simulink model "ChiefMaster_TTC580"  (R2022b)
settings: Solver=FixedStepAuto  StartTime=0.0  StopTime=10  FixedStep=0.01  RelTol=1e-3
values from neighbouring files (symbols this model uses):
  BattBox1_No = single(1)    [Parameters.m]
  BattBox2_No = single(2)    [Parameters.m]
  BattBox3_No = single(3)    [Parameters.m]
  CurrentLB = single(-3)    [Parameters.m]
  CurrentReductionConstant_Lvl0 = single(0.03)    [Parameters.m]
  CurrentReductionConstant_Lvl1 = single(0.05)    [Parameters.m]
  CurrentReductionConstant_Lvl2 = single(0.07)    [Parameters.m]
  CurrentReductionConstant_Lvl3 = single(0.1)    [Parameters.m]
  CurrentUB = single(3)    [Parameters.m]
  DCHV_Minus_In_Delay_ms = single(500)    [Parameters.m]
  FL_sHVC_CellBalanceVoltage_mV = single(3500)    [Parameters.m]
  FL_sInrushCurrent_dividebyzero = single(0.00001)    [Parameters.m]
  FL_u8HMI_BuzzerTimer = uint8(3)    [Parameters.m]
  IP_boActValue = true    [Parameters.m]
  IP_boDeactValue = false    [Parameters.m]
  IP_boInitValue = false    [Parameters.m]
  IP_s_LB = 18000    [Parameters.m]
  IP_s_UB = 22000    [Parameters.m]
  IP_sBatt1_ChargeCurrentMax_Factor = single(0.1)    [Parameters.m]
  IP_sBatt1_ChargeCurrentMax_LB = single(0)    [Parameters.m]
  IP_sBatt1_ChargeCurrentMax_Offset = single(0)    [Parameters.m]
  IP_sBatt1_ChargeCurrentMax_UB = single(6553.5)    [Parameters.m]
  IP_sBatt1_Current_Factor = single(0.1)    [Parameters.m]
  IP_sBatt1_Current_LB = single(-3276.8)    [Parameters.m]
  IP_sBatt1_Current_Offset = single(0)    [Parameters.m]
  IP_sBatt1_Current_UB = single(3276.8)    [Parameters.m]
  IP_sBatt1_DisChargeCurrentMax_Factor = single(0.1)    [Parameters.m]
  IP_sBatt1_DisChargeCurrentMax_LB = single(0)    [Parameters.m]
  IP_sBatt1_DisChargeCurrentMax_Offset = single(0)    [Parameters.m]
  IP_sBatt1_DisChargeCurrentMax_UB = single(6553.5)    [Parameters.m]
  IP_sBatt1_InsulationResistance_Factor = single(5)    [Parameters.m]
  IP_sBatt1_InsulationResistance_LB = single(0)    [Parameters.m]
  IP_sBatt1_InsulationResistance_Offset = single(0)    [Parameters.m]
  IP_sBatt1_InsulationResistance_UB = single(0)    [Parameters.m]
  IP_sBatt1_LiBa_IntResist_mOhm = single(25)    [Parameters.m]
  IP_sBatt1_SOC_Factor = single(1)    [Parameters.m]
  IP_sBatt1_SOC_LB = single(0)    [Parameters.m]
  IP_sBatt1_SOC_Offset = single(0)    [Parameters.m]
  IP_sBatt1_SOC_UB = single(100)    [Parameters.m]
  IP_sBatt1_SOH_Factor = single(1)    [Parameters.m]
  IP_sBatt1_SOH_LB = single(0)    [Parameters.m]
  IP_sBatt1_SOH_Offset = single(0)    [Parameters.m]
  IP_sBatt1_SOH_UB = single(100)    [Parameters.m]
  IP_sBatt1_Ubatt_Factor = single(0.1)    [Parameters.m]
  IP_sBatt1_Ubatt_LB = single(0)    [Parameters.m]
  IP_sBatt1_Ubatt_Offset = single(0)    [Parameters.m]
  IP_sBatt1_Ubatt_UB = single(6553.5)    [Parameters.m]
  IP_sBatt1_UserRi_Factor = single(1)    [Parameters.m]
  IP_sBatt1_UserRi_LB = single(0)    [Parameters.m]
  IP_sBatt1_UserRi_Offset = single(0)    [Parameters.m]
  IP_sBatt1_UserRi_UB = single(255)    [Parameters.m]
  IP_sBatt1_VoltageAtSensor_Factor = single(0.02)    [Parameters.m]
  IP_sBatt1_VoltageAtSensor_LB = single(0)    [Parameters.m]
  IP_sBatt1_VoltageAtSensor_Offset = single(0)    [Parameters.m]
  IP_sBatt1_VoltageAtSensor_UB = single(1310.7)    [Parameters.m]
  IP_sBatt2_LiBa_IntResist_mOhm = single(25)    [Parameters.m]
  IP_sBatt3_LiBa_IntResist_mOhm = single(25)    [Parameters.m]
  IP_sEM_LB = 2000    [Parameters.m]
  IP_sEM_UB = 8000    [Parameters.m]
  IP_sFB_LB = 5000    [Parameters.m]
  IP_sFB_UB = 10000    [Parameters.m]
  IP_sHVIL_LB = 12000    [Parameters.m]
  IP_sHVIL_UB = 15000    [Parameters.m]
  IP_sLoad_Voltage_Factor = single(1)    [Parameters.m]
  IP_sLoad_Voltage_LB = single(0)    [Parameters.m]
  IP_sLoad_Voltage_Offset = single(0)    [Parameters.m]
  IP_sLoad_Voltage_UB = single(65535)    [Parameters.m]
  IP_u8HVIL_Delay_ms = uint8(100)    [Parameters.m]
  IP_u8HW_IN_delay_ms = uint8(100)    [Parameters.m]
  IT_sInsulationSafeValue_kOhm = single(650)    [Parameters.m]
  IT_u8IMD_DelayTime_s = uint8(20)    [Parameters.m]
  MainHV_Minus_In_Delay = single(5)    [Parameters.m]
  MainHV_StatusDelay = single(5)    [Parameters.m]
  NotAvailable_uint16 = single(65535)    [Parameters.m]
  NotAvailable_uint8 = uint8(255)    [Parameters.m]
  OP_boHVIL_Supply = boolean(1)    [Parameters.m]
  SafeCurrentToCloseHV_A = single(5)    [Parameters.m]
  SafeVoltageToCloseHV_V = single(0.5)    [Parameters.m]
  UnexpectedBattChargingFcn_Available = boolean(1)    [Parameters.m]
  Voltage_NA_UB = uint16(65535)    [Parameters.m]
  VoltageSensorAvailableBB1 = boolean(0)    [Parameters.m]
  VoltageSensorAvailableBB2 = boolean(0)    [Parameters.m]
  VoltageSensorAvailableBB3 = boolean(0)    [Parameters.m]
libraries: simulink x184, Library_DataProcessing_v1_1 x167, Library_DataProcessing_v1 x142, libCM x28
(part 2 of 19)

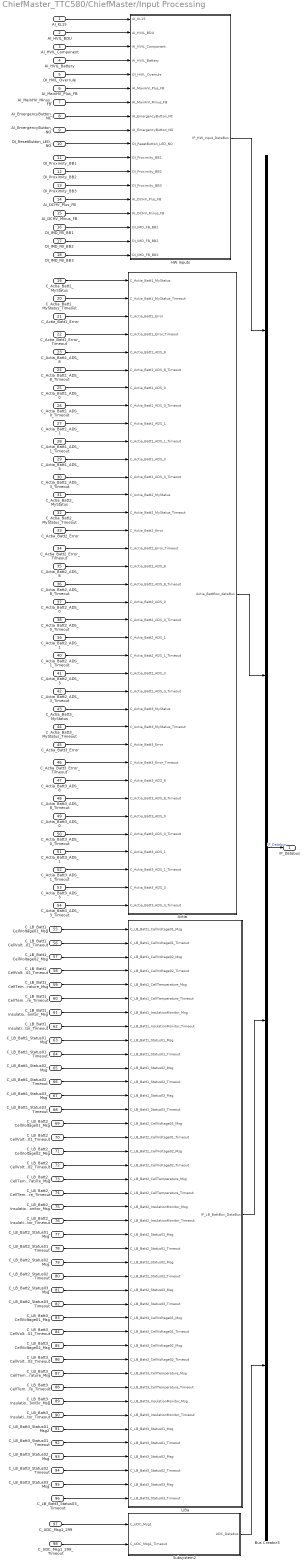
== system ChiefMaster_TTC580/ChiefMaster/Input Processing ==
  AI_KL15 : Inport  OutDataTypeStr=single
  AI_HVIL_BDU : Inport  Port=2  OutDataTypeStr=single
  AI_HVIL_Component : Inport  Port=3  OutDataTypeStr=single
  AI_HVIL_Battery : Inport  Port=4  OutDataTypeStr=single
  DI_HVIL_Overrule : Inport  Port=5  OutDataTypeStr=boolean
  AI_MainHV_Plus_FB : Inport  Port=6  OutDataTypeStr=single
  AI_MainHV_Minus_FB : Inport  Port=7  OutDataTypeStr=single
  AI_EmergencyButton_NC : Inport  Port=8  OutDataTypeStr=single
  AI_EmergencyButton_NO : Inport  Port=9
  DI_ResetButton_LED_NO : Inport  Port=10
  DI_Proximity_BB1 : Inport  Port=11
  DI_Proximity_BB2 : Inport  Port=12
  DI_Proximity_BB3 : Inport  Port=13
  AI_DCHV_Plus_FB : Inport  Port=14  OutDataTypeStr=single
  AI_DCHV_Minus_FB : Inport  Port=15  OutDataTypeStr=single
  DI_IMD_FB_BB1 : Inport  Port=16
  DI_IMD_FB_BB2 : Inport  Port=17
  DI_IMD_FB_BB3 : Inport  Port=18
  C_Actia_Batt1_MyStatus : Inport  Port=19  OutDataTypeStr=uint8
  C_Actia_Batt1_MyStatus_Timeout : Inport  Port=20  OutDataTypeStr=boolean
  C_Actia_Batt1_Error : Inport  Port=21  OutDataTypeStr=uint8
  C_Actia_Batt1_Error_Timeout : Inport  Port=22  OutDataTypeStr=boolean
  C_Actia_Batt1_ADS_8 : Inport  Port=23  OutDataTypeStr=uint8
  C_Actia_Batt1_ADS_8_Timeout : Inport  Port=24  OutDataTypeStr=boolean
  C_Actia_Batt1_ADS_0 : Inport  Port=25
  C_Actia_Batt1_ADS_0_Timeout : Inport  Port=26
  C_Actia_Batt1_ADS_1 : Inport  Port=27  OutDataTypeStr=uint8
  C_Actia_Batt1_ADS_1_Timeout : Inport  Port=28  OutDataTypeStr=boolean
  C_Actia_Batt1_ADS_3 : Inport  Port=29  OutDataTypeStr=uint8
  C_Actia_Batt1_ADS_3_Timeout : Inport  Port=30  OutDataTypeStr=boolean
  C_Actia_Batt2_MyStatus : Inport  Port=31  OutDataTypeStr=uint8
  C_Actia_Batt2_MyStatus_Timeout : Inport  Port=32  OutDataTypeStr=boolean
  C_Actia_Batt2_Error : Inport  Port=33  OutDataTypeStr=uint8
  C_Actia_Batt2_Error_Timeout : Inport  Port=34  OutDataTypeStr=boolean
  C_Actia_Batt2_ADS_8 : Inport  Port=35  OutDataTypeStr=uint8
  C_Actia_Batt2_ADS_8_Timeout : Inport  Port=36  OutDataTypeStr=boolean
  C_Actia_Batt2_ADS_0 : Inport  Port=37
  C_Actia_Batt2_ADS_0_Timeout : Inport  Port=38
  C_Actia_Batt2_ADS_1 : Inport  Port=39  OutDataTypeStr=uint8
  C_Actia_Batt2_ADS_1_Timeout : Inport  Port=40  OutDataTypeStr=boolean
  C_Actia_Batt2_ADS_3 : Inport  Port=41  OutDataTypeStr=uint8
  C_Actia_Batt2_ADS_3_Timeout : Inport  Port=42  OutDataTypeStr=boolean
  C_Actia_Batt3_MyStatus : Inport  Port=43  OutDataTypeStr=uint8
  C_Actia_Batt3_MyStatus_Timeout : Inport  Port=44  OutDataTypeStr=boolean
  C_Actia_Batt3_Error : Inport  Port=45  OutDataTypeStr=uint8
  C_Actia_Batt3_Error_Timeout : Inport  Port=46  OutDataTypeStr=boolean
  C_Actia_Batt3_ADS_8 : Inport  Port=47  OutDataTypeStr=uint8
  C_Actia_Batt3_ADS_8_Timeout : Inport  Port=48  OutDataTypeStr=boolean
  C_Actia_Batt3_ADS_0 : Inport  Port=49
  C_Actia_Batt3_ADS_0_Timeout : Inport  Port=50
  C_Actia_Batt3_ADS_1 : Inport  Port=51  OutDataTypeStr=uint8
  C_Actia_Batt3_ADS_1_Timeout : Inport  Port=52  OutDataTypeStr=boolean
  C_Actia_Batt3_ADS_3 : Inport  Port=53  OutDataTypeStr=uint8
  C_Actia_Batt3_ADS_3_Timeout : Inport  Port=54  OutDataTypeStr=boolean
  C_LB_Batt1_CellVoltage01_Msg : Inport  Port=55
  C_LB_Batt1_CellVoltage01_Timeout : Inport  Port=56
  C_LB_Batt1_CellVoltage02_Msg : Inport  Port=57
  C_LB_Batt1_CellVoltage02_Timeout : Inport  Port=58
  C_LB_Batt1_CellTemperature_Msg : Inport  Port=59
  C_LB_Batt1_CellTemperature_Timeout : Inport  Port=60
  C_LB_Batt1_InsulationMonitor_Msg : Inport  Port=61
  C_LB_Batt1_InsulationMonitor_Timeout : Inport  Port=62
  C_LB_Batt1_Status01_Msg : Inport  Port=63
  C_LB_Batt1_Status01_Timeout : Inport  Port=64
  C_LB_Batt1_Status02_Msg : Inport  Port=65
  C_LB_Batt1_Status02_Timeout : Inport  Port=66
  C_LB_Batt1_Status03_Msg : Inport  Port=67
  C_LB_Batt1_Status03_Timeout : Inport  Port=68
  C_LB_Batt2_CellVoltage01_Msg : Inport  Port=69
  C_LB_Batt2_CellVoltage01_Timeout : Inport  Port=70
  C_LB_Batt2_CellVoltage02_Msg : Inport  Port=71
  C_LB_Batt2_CellVoltage02_Timeout : Inport  Port=72
  C_LB_Batt2_CellTemperature_Msg : Inport  Port=73
  C_LB_Batt2_CellTemperature_Timeout : Inport  Port=74
  C_LB_Batt2_InsulationMonitor_Msg : Inport  Port=75
  C_LB_Batt2_InsulationMonitor_Timeout : Inport  Port=76
  C_LB_Batt2_Status01_Msg : Inport  Port=77
  C_LB_Batt2_Status01_Timeout : Inport  Port=78
  C_LB_Batt2_Status02_Msg : Inport  Port=79
  C_LB_Batt2_Status02_Timeout : Inport  Port=80
  C_LB_Batt2_Status03_Msg : Inport  Port=81
  C_LB_Batt2_Status03_Timeout : Inport  Port=82
  C_LB_Batt3_CellVoltage01_Msg : Inport  Port=83
  C_LB_Batt3_CellVoltage01_Timeout : Inport  Port=84
  C_LB_Batt3_CellVoltage02_Msg : Inport  Port=85
  C_LB_Batt3_CellVoltage02_Timeout : Inport  Port=86
  C_LB_Batt3_CellTemperature_Msg : Inport  Port=87
  C_LB_Batt3_CellTemperature_Timeout : Inport  Port=88
  C_LB_Batt3_InsulationMonitor_Msg : Inport  Port=89
  C_LB_Batt3_InsulationMonitor_Timeout : Inport  Port=90
  C_LB_Batt3_Status01_Msg2 : Inport  Port=91
  C_LB_Batt3_Status01_Timeout : Inport  Port=92
  C_LB_Batt3_Status02_Msg : Inport  Port=93
  C_LB_Batt3_Status02_Timeout : Inport  Port=94
  C_LB_Batt3_Status03_Msg : Inport  Port=95
  C_LB_Batt3_Status03_Timeout : Inport  Port=96
  C_UDC_Msg1_299 : Inport  Port=97
  C_UDC_Msg1_299_Timeout : Inport  Port=98
  Actia : Subsystem
  Bus Creator3 : BusCreator  Inputs=4
  HW Inputs : Subsystem
  LiBa : Subsystem
  Subsystem2 : Subsystem
  IP_Databus : Outport
  wires:
  AI_MainHV_Minus_FB/1 -> HW Inputs/7(AI_MainHV_Minus_FB)
  AI_KL15/1 -> HW Inputs/1(AI_KL15)
  AI_MainHV_Plus_FB/1 -> HW Inputs/6(AI_MainHV_Plus_FB)
  Bus Creator3/1 -> IP_Databus/1  "IP_Databus"
  Subsystem2/1(UDC_Databus) -> Bus Creator3/4
  C_LB_Batt1_CellVoltage02_Msg/1 -> LiBa/3(C_LB_Batt1_CellVoltage02_Msg)
  C_LB_Batt1_CellVoltage01_Timeout/1 -> LiBa/2(C_LB_Batt1_CellVoltage01_Timeout)
  C_LB_Batt1_CellVoltage01_Msg/1 -> LiBa/1(C_LB_Batt1_CellVoltage01_Msg)
  C_LB_Batt1_InsulationMonitor_Msg/1 -> LiBa/7(C_LB_Batt1_InsulationMonitor_Msg)
  C_LB_Batt1_CellTemperature_Timeout/1 -> LiBa/6(C_LB_Batt1_CellTemperature_Timeout)
  C_LB_Batt1_CellTemperature_Msg/1 -> LiBa/5(C_LB_Batt1_CellTemperature_Msg)
  C_LB_Batt1_CellVoltage02_Timeout/1 -> LiBa/4(C_LB_Batt1_CellVoltage02_Timeout)
  C_UDC_Msg1_299/1 -> Subsystem2/1(C_UDC_Msg1)
  C_LB_Batt1_Status02_Msg/1 -> LiBa/11(C_LB_Batt1_Status02_Msg)
  C_LB_Batt1_Status01_Timeout/1 -> LiBa/10(C_LB_Batt1_Status01_Timeout)
  C_LB_Batt1_Status01_Msg/1 -> LiBa/9(C_LB_Batt1_Status01_Msg)
  C_LB_Batt1_InsulationMonitor_Timeout/1 -> LiBa/8(C_LB_Batt1_InsulationMonitor_Timeout)
  C_LB_Batt1_Status03_Timeout/1 -> LiBa/14(C_LB_Batt1_Status03_Timeout)
  C_LB_Batt1_Status03_Msg/1 -> LiBa/13(C_LB_Batt1_Status03_Msg)
  C_LB_Batt1_Status02_Timeout/1 -> LiBa/12(C_LB_Batt1_Status02_Timeout)
  C_UDC_Msg1_299_Timeout/1 -> Subsystem2/2(C_UDC_Msg1_Timeout)
  HW Inputs/1(IP_HW_Input_DataBus) -> Bus Creator3/1
  Actia/1(Actia_BattBox_dataBus) -> Bus Creator3/2
  C_LB_Batt3_Status03_Timeout/1 -> LiBa/42(C_LB_Batt3_Status03_Timeout)
  C_LB_Batt3_CellVoltage02_Msg/1 -> LiBa/31(C_LB_Batt3_CellVoltage02_Msg)
  C_LB_Batt3_InsulationMonitor_Timeout/1 -> LiBa/36(C_LB_Batt3_InsulationMonitor_Timeout)
  C_LB_Batt3_CellVoltage02_Timeout/1 -> LiBa/32(C_LB_Batt3_CellVoltage02_Timeout)
  C_LB_Batt3_CellVoltage01_Timeout/1 -> LiBa/30(C_LB_Batt3_CellVoltage01_Timeout)
  C_LB_Batt3_Status01_Msg2/1 -> LiBa/37(C_LB_Batt3_Status01_Msg)
  C_LB_Batt3_Status02_Timeout/1 -> LiBa/40(C_LB_Batt3_Status02_Timeout)
  C_LB_Batt3_Status02_Msg/1 -> LiBa/39(C_LB_Batt3_Status02_Msg)
  C_LB_Batt3_CellTemperature_Timeout/1 -> LiBa/34(C_LB_Batt3_CellTemperature_Timeout)
  C_LB_Batt3_Status03_Msg/1 -> LiBa/41(C_LB_Batt3_Status03_Msg)
  C_LB_Batt3_CellTemperature_Msg/1 -> LiBa/33(C_LB_Batt3_CellTemperature_Msg)
  C_LB_Batt3_InsulationMonitor_Msg/1 -> LiBa/35(C_LB_Batt3_InsulationMonitor_Msg)
  C_LB_Batt2_Status02_Timeout/1 -> LiBa/26(C_LB_Batt2_Status02_Timeout)
  C_LB_Batt2_Status03_Timeout/1 -> LiBa/28(C_LB_Batt2_Status03_Timeout)
  C_LB_Batt3_Status01_Timeout/1 -> LiBa/38(C_LB_Batt3_Status01_Timeout)
  C_LB_Batt2_Status03_Msg/1 -> LiBa/27(C_LB_Batt2_Status03_Msg)
  C_LB_Batt2_Status01_Timeout/1 -> LiBa/24(C_LB_Batt2_Status01_Timeout)
  C_LB_Batt2_Status01_Msg/1 -> LiBa/23(C_LB_Batt2_Status01_Msg)
  C_LB_Batt2_InsulationMonitor_Timeout/1 -> LiBa/22(C_LB_Batt2_InsulationMonitor_Timeout)
  C_LB_Batt2_CellVoltage02_Msg/1 -> LiBa/17(C_LB_Batt2_CellVoltage02_Msg)
  C_LB_Batt2_CellVoltage01_Timeout/1 -> LiBa/16(C_LB_Batt2_CellVoltage01_Timeout)
  C_LB_Batt2_InsulationMonitor_Msg/1 -> LiBa/21(C_LB_Batt2_InsulationMonitor_Msg)
  C_LB_Batt2_CellTemperature_Timeout/1 -> LiBa/20(C_LB_Batt2_CellTemperature_Timeout)
  C_LB_Batt2_CellVoltage02_Timeout/1 -> LiBa/18(C_LB_Batt2_CellVoltage02_Timeout)
  C_LB_Batt2_Status02_Msg/1 -> LiBa/25(C_LB_Batt2_Status02_Msg)
  C_LB_Batt2_CellTemperature_Msg/1 -> LiBa/19(C_LB_Batt2_CellTemperature_Msg)
  C_LB_Batt2_CellVoltage01_Msg/1 -> LiBa/15(C_LB_Batt2_CellVoltage01_Msg)
  C_LB_Batt3_CellVoltage01_Msg/1 -> LiBa/29(C_LB_Batt3_CellVoltage01_Msg)
  LiBa/1(IP_LB_BattBox_DataBus) -> Bus Creator3/3
  AI_HVIL_Battery/1 -> HW Inputs/4(AI_HVIL_Battery)
  AI_HVIL_Component/1 -> HW Inputs/3(AI_HVIL_Component)
  AI_HVIL_BDU/1 -> HW Inputs/2(AI_HVIL_BDU)
  AI_EmergencyButton_NC/1 -> HW Inputs/8(AI_EmergencyButton_NC)
  AI_EmergencyButton_NO/1 -> HW Inputs/9(AI_EmergencyButton_NO)
  DI_ResetButton_LED_NO/1 -> HW Inputs/10(DI_ResetButton_LED_NO)
  DI_Proximity_BB1/1 -> HW Inputs/11(DI_Proximity_BB1)
  DI_Proximity_BB2/1 -> HW Inputs/12(DI_Proximity_BB2)
  DI_Proximity_BB3/1 -> HW Inputs/13(DI_Proximity_BB3)
  AI_DCHV_Plus_FB/1 -> HW Inputs/14(AI_DCHV_Plus_FB)
  AI_DCHV_Minus_FB/1 -> HW Inputs/15(AI_DCHV_Minus_FB)
  C_Actia_Batt1_MyStatus/1 -> Actia/1(C_Actia_Batt1_MyStatus)
  C_Actia_Batt1_MyStatus_Timeout/1 -> Actia/2(C_Actia_Batt1_MyStatus_Timeout)
  C_Actia_Batt1_Error/1 -> Actia/3(C_Actia_Batt1_Error)
  C_Actia_Batt1_Error_Timeout/1 -> Actia/4(C_Actia_Batt1_Error_Timeout)
  C_Actia_Batt1_ADS_8/1 -> Actia/5(C_Actia_Batt1_ADS_8)
  C_Actia_Batt1_ADS_8_Timeout/1 -> Actia/6(C_Actia_Batt1_ADS_8_Timeout)
  C_Actia_Batt1_ADS_1/1 -> Actia/9(C_Actia_Batt1_ADS_1)
  C_Actia_Batt1_ADS_1_Timeout/1 -> Actia/10(C_Actia_Batt1_ADS_1_Timeout)
  C_Actia_Batt1_ADS_3/1 -> Actia/11(C_Actia_Batt1_ADS_3)
  C_Actia_Batt1_ADS_3_Timeout/1 -> Actia/12(C_Actia_Batt1_ADS_3_Timeout)
  C_Actia_Batt2_MyStatus/1 -> Actia/13(C_Actia_Batt2_MyStatus)
  C_Actia_Batt2_MyStatus_Timeout/1 -> Actia/14(C_Actia_Batt2_MyStatus_Timeout)
  C_Actia_Batt2_Error/1 -> Actia/15(C_Actia_Batt2_Error)
  C_Actia_Batt2_Error_Timeout/1 -> Actia/16(C_Actia_Batt2_Error_Timeout)
  C_Actia_Batt2_ADS_8/1 -> Actia/17(C_Actia_Batt2_ADS_8)
  C_Actia_Batt2_ADS_8_Timeout/1 -> Actia/18(C_Actia_Batt2_ADS_8_Timeout)
  C_Actia_Batt2_ADS_1/1 -> Actia/21(C_Actia_Batt2_ADS_1)
  C_Actia_Batt2_ADS_1_Timeout/1 -> Actia/22(C_Actia_Batt2_ADS_1_Timeout)
  C_Actia_Batt2_ADS_3/1 -> Actia/23(C_Actia_Batt2_ADS_3)
  C_Actia_Batt2_ADS_3_Timeout/1 -> Actia/24(C_Actia_Batt2_ADS_3_Timeout)
  C_Actia_Batt3_MyStatus/1 -> Actia/25(C_Actia_Batt3_MyStatus)
  C_Actia_Batt3_MyStatus_Timeout/1 -> Actia/26(C_Actia_Batt3_MyStatus_Timeout)
  C_Actia_Batt3_Error/1 -> Actia/27(C_Actia_Batt3_Error)
  C_Actia_Batt3_Error_Timeout/1 -> Actia/28(C_Actia_Batt3_Error_Timeout)
  C_Actia_Batt3_ADS_8/1 -> Actia/29(C_Actia_Batt3_ADS_8)
  C_Actia_Batt3_ADS_8_Timeout/1 -> Actia/30(C_Actia_Batt3_ADS_8_Timeout)
  C_Actia_Batt3_ADS_1/1 -> Actia/33(C_Actia_Batt3_ADS_1)
  C_Actia_Batt3_ADS_1_Timeout/1 -> Actia/34(C_Actia_Batt3_ADS_1_Timeout)
  C_Actia_Batt3_ADS_3/1 -> Actia/35(C_Actia_Batt3_ADS_3)
  C_Actia_Batt3_ADS_3_Timeout/1 -> Actia/36(C_Actia_Batt3_ADS_3_Timeout)
  C_Actia_Batt1_ADS_0_Timeout/1 -> Actia/8(C_Actia_Batt1_ADS_0_Timeout)
  C_Actia_Batt1_ADS_0/1 -> Actia/7(C_Actia_Batt1_ADS_0)
  C_Actia_Batt2_ADS_0/1 -> Actia/19(C_Actia_Batt2_ADS_0)
  C_Actia_Batt2_ADS_0_Timeout/1 -> Actia/20(C_Actia_Batt2_ADS_0_Timeout)
  C_Actia_Batt3_ADS_0_Timeout/1 -> Actia/32(C_Actia_Batt3_ADS_0_Timeout)
  C_Actia_Batt3_ADS_0/1 -> Actia/31(C_Actia_Batt3_ADS_0)
  DI_HVIL_Overrule/1 -> HW Inputs/5(DI_HVIL_Overrule)
  DI_IMD_FB_BB1/1 -> HW Inputs/16(DI_IMD_FB_BB1)
  DI_IMD_FB_BB2/1 -> HW Inputs/17(DI_IMD_FB_BB2)
  DI_IMD_FB_BB3/1 -> HW Inputs/18(DI_IMD_FB_BB3)

== system ChiefMaster_TTC580/ChiefMaster/Input Translation ==
  IP_Databus : Inport
  IMD_Req_Databus : Inport  Port=2
  Battery Selection : Subsystem
      settings: RTWFcnNameOpts=Use subsystem name  RTWFileNameOpts=Use subsystem name
  Battery Signals : Subsystem
  Bus Creator : BusCreator  Inputs=4
  HW Inputs : Subsystem
  UDC : Subsystem
  IT_Databus : Outport
  wires:
  IMD_Req_Databus/1 -> Battery Signals/2(IMD_Req_Databus)
  Battery Signals/1(IT_BatterySignal_Databus) -> Bus Creator/3
  Bus Creator/1 -> IT_Databus/1  "IT_Databus"
  HW Inputs/1(IT_HW_Input_Databus) -> Bus Creator/2
  UDC/1(IT_UDC_Databus) -> Bus Creator/4
  IP_Databus/1 -> UDC/1(IP_Databus), Battery Signals/1(IP_Databus), Battery Selection/1(IP_Databus), HW Inputs/1(IP_Databus)
  Battery Selection/1(IT_SelectBattery_Databus) -> Bus Creator/1

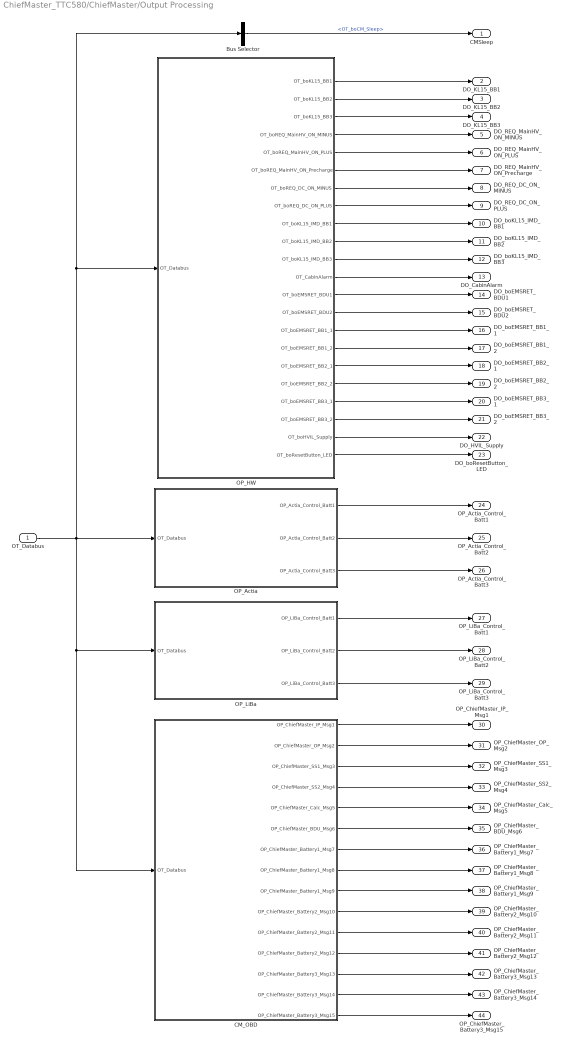
== system ChiefMaster_TTC580/ChiefMaster/Output Processing ==
  OT_Databus : Inport
  Bus Selector : BusSelector  OutputSignals=OT_boCM_Sleep
  CM_OBD : Subsystem
  OP_Actia : Subsystem
  OP_HW : Subsystem
  OP_LiBa : Subsystem
  CMSleep : Outport
  DO_KL15_BB1 : Outport  Port=2
  DO_KL15_BB2 : Outport  Port=3
  DO_KL15_BB3 : Outport  Port=4
  DO_REQ_MainHV_ON_MINUS : Outport  Port=5
  DO_REQ_MainHV_ON_PLUS : Outport  Port=6
  DO_REQ_MainHV_ON_Precharge : Outport  Port=7
  DO_REQ_DC_ON_MINUS : Outport  Port=8
  DO_REQ_DC_ON_PLUS : Outport  Port=9
  DO_boKL15_IMD_BB1 : Outport  Port=10
  DO_boKL15_IMD_BB2 : Outport  Port=11
  DO_boKL15_IMD_BB3 : Outport  Port=12
  DO_CabinAlarm : Outport  Port=13
  DO_boEMSRET_BDU1 : Outport  Port=14  OutDataTypeStr=boolean
  DO_boEMSRET_BDU2 : Outport  Port=15  OutDataTypeStr=boolean
  DO_boEMSRET_BB1_1 : Outport  Port=16  OutDataTypeStr=boolean
  DO_boEMSRET_BB1_2 : Outport  Port=17  OutDataTypeStr=boolean
  DO_boEMSRET_BB2_1 : Outport  Port=18  OutDataTypeStr=boolean
  DO_boEMSRET_BB2_2 : Outport  Port=19  OutDataTypeStr=boolean
  DO_boEMSRET_BB3_1 : Outport  Port=20  OutDataTypeStr=boolean
  DO_boEMSRET_BB3_2 : Outport  Port=21  OutDataTypeStr=boolean
  DO_HVIL_Supply : Outport  Port=22  OutDataTypeStr=boolean
  DO_boResetButton_LED : Outport  Port=23  OutDataTypeStr=boolean
  OP_Actia_Control_Batt1 : Outport  Port=24
  OP_Actia_Control_Batt2 : Outport  Port=25
  OP_Actia_Control_Batt3 : Outport  Port=26
  OP_LiBa_Control_Batt1 : Outport  Port=27
  OP_LiBa_Control_Batt2 : Outport  Port=28
  OP_LiBa_Control_Batt3 : Outport  Port=29
  OP_ChiefMaster_IP_Msg1 : Outport  Port=30
  OP_ChiefMaster_OP_Msg2 : Outport  Port=31
  OP_ChiefMaster_SS1_Msg3 : Outport  Port=32
  OP_ChiefMaster_SS2_Msg4 : Outport  Port=33
  OP_ChiefMaster_Calc_Msg5 : Outport  Port=34
  OP_ChiefMaster_BDU_Msg6 : Outport  Port=35
  OP_ChiefMaster_Battery1_Msg7 : Outport  Port=36
  OP_ChiefMaster_Battery1_Msg8 : Outport  Port=37
  OP_ChiefMaster_Battery1_Msg9 : Outport  Port=38
  OP_ChiefMaster_Battery2_Msg10 : Outport  Port=39
  OP_ChiefMaster_Battery2_Msg11 : Outport  Port=40
  OP_ChiefMaster_Battery2_Msg12 : Outport  Port=41
  OP_ChiefMaster_Battery3_Msg13 : Outport  Port=42
  OP_ChiefMaster_Battery3_Msg14 : Outport  Port=43
  OP_ChiefMaster_Battery3_Msg15 : Outport  Port=44
  wires:
  OT_Databus/1 -> CM_OBD/1(OT_Databus), OP_LiBa/1(OT_Databus), Bus Selector/1, OP_HW/1(OT_Databus), OP_Actia/1(OT_Databus)
  OP_Actia/1(OP_Actia_Control_Batt1) -> OP_Actia_Control_Batt1/1
  OP_Actia/2(OP_Actia_Control_Batt2) -> OP_Actia_Control_Batt2/1
  OP_Actia/3(OP_Actia_Control_Batt3) -> OP_Actia_Control_Batt3/1
  OP_LiBa/1(OP_LiBa_Control_Batt1) -> OP_LiBa_Control_Batt1/1
  OP_LiBa/2(OP_LiBa_Control_Batt2) -> OP_LiBa_Control_Batt2/1
  OP_LiBa/3(OP_LiBa_Control_Batt3) -> OP_LiBa_Control_Batt3/1
  OP_HW/1(OT_boKL15_BB1) -> DO_KL15_BB1/1
  OP_HW/2(OT_boKL15_BB2) -> DO_KL15_BB2/1
  OP_HW/3(OT_boKL15_BB3) -> DO_KL15_BB3/1
  OP_HW/4(OT_boREQ_MainHV_ON_MINUS) -> DO_REQ_MainHV_ON_MINUS/1
  OP_HW/5(OT_boREQ_MainHV_ON_PLUS) -> DO_REQ_MainHV_ON_PLUS/1
  OP_HW/6(OT_boREQ_MainHV_ON_Precharge) -> DO_REQ_MainHV_ON_Precharge/1
  Bus Selector/1 -> CMSleep/1  "<OT_boCM_Sleep>"
  CM_OBD/1(OP_ChiefMaster_IP_Msg1) -> OP_ChiefMaster_IP_Msg1/1
  CM_OBD/2(OP_ChiefMaster_OP_Msg2) -> OP_ChiefMaster_OP_Msg2/1
  CM_OBD/3(OP_ChiefMaster_SS1_Msg3) -> OP_ChiefMaster_SS1_Msg3/1
  CM_OBD/4(OP_ChiefMaster_SS2_Msg4) -> OP_ChiefMaster_SS2_Msg4/1
  CM_OBD/5(OP_ChiefMaster_Calc_Msg5) -> OP_ChiefMaster_Calc_Msg5/1
  CM_OBD/6(OP_ChiefMaster_BDU_Msg6) -> OP_ChiefMaster_BDU_Msg6/1
  CM_OBD/7(OP_ChiefMaster_Battery1_Msg7) -> OP_ChiefMaster_Battery1_Msg7/1
  CM_OBD/8(OP_ChiefMaster_Battery1_Msg8) -> OP_ChiefMaster_Battery1_Msg8/1
  CM_OBD/10(OP_ChiefMaster_Battery2_Msg10) -> OP_ChiefMaster_Battery2_Msg10/1
  CM_OBD/11(OP_ChiefMaster_Battery2_Msg11) -> OP_ChiefMaster_Battery2_Msg11/1
  CM_OBD/13(OP_ChiefMaster_Battery3_Msg13) -> OP_ChiefMaster_Battery3_Msg13/1
  CM_OBD/14(OP_ChiefMaster_Battery3_Msg14) -> OP_ChiefMaster_Battery3_Msg14/1
  OP_HW/7(OT_boREQ_DC_ON_MINUS) -> DO_REQ_DC_ON_MINUS/1
  OP_HW/8(OT_boREQ_DC_ON_PLUS) -> DO_REQ_DC_ON_PLUS/1
  CM_OBD/9(OP_ChiefMaster_Battery1_Msg9) -> OP_ChiefMaster_Battery1_Msg9/1
  CM_OBD/12(OP_ChiefMaster_Battery2_Msg12) -> OP_ChiefMaster_Battery2_Msg12/1
  CM_OBD/15(OP_ChiefMaster_Battery3_Msg15) -> OP_ChiefMaster_Battery3_Msg15/1
  OP_HW/9(OT_boKL15_IMD_BB1) -> DO_boKL15_IMD_BB1/1
  OP_HW/10(OT_boKL15_IMD_BB2) -> DO_boKL15_IMD_BB2/1
  OP_HW/11(OT_boKL15_IMD_BB3) -> DO_boKL15_IMD_BB3/1
  OP_HW/12(OT_CabinAlarm) -> DO_CabinAlarm/1
  OP_HW/13(OT_boEMSRET_BDU1) -> DO_boEMSRET_BDU1/1
  OP_HW/14(OT_boEMSRET_BDU2) -> DO_boEMSRET_BDU2/1
  OP_HW/15(OT_boEMSRET_BB1_1) -> DO_boEMSRET_BB1_1/1
  OP_HW/16(OT_boEMSRET_BB1_2) -> DO_boEMSRET_BB1_2/1
  OP_HW/17(OT_boEMSRET_BB2_1) -> DO_boEMSRET_BB2_1/1
  OP_HW/18(OT_boEMSRET_BB2_2) -> DO_boEMSRET_BB2_2/1
  OP_HW/19(OT_boEMSRET_BB3_1) -> DO_boEMSRET_BB3_1/1
  OP_HW/20(OT_boEMSRET_BB3_2) -> DO_boEMSRET_BB3_2/1
  OP_HW/21(OT_boHVIL_Supply) -> DO_HVIL_Supply/1
  OP_HW/22(OT_boResetButton_LED) -> DO_boResetButton_LED/1

== system ChiefMaster_TTC580/ChiefMaster/Output Translation ==
  FL_Databus : Inport
  BDUControl : Subsystem
  BatteryBox : Subsystem
  Bus Creator : BusCreator  Inputs=7
  Bus Selector : BusSelector  OutputSignals=FL_KL15_Databus.FL_boCMSleep
  IMD : Subsystem
  KL15 : Subsystem
  Signal Copy : SignalConversion  OverrideOpt=off
  SystemStatus : Subsystem
  OT_Databus : Outport
  wires:
  FL_Databus/1 -> Bus Creator/1, Bus Selector/1, KL15/1(FL_Databus), SystemStatus/1(FL_Databus), BDUControl/1(FL_Databus), BatteryBox/1(FL_Databus), IMD/1(FL_Databus)
  KL15/1(OT_KL15_Databus) -> Bus Creator/3
  Bus Creator/1 -> OT_Databus/1
  IMD/1(OT_IMD_Databus) -> Bus Creator/4
  BatteryBox/1(OT_BatteryBox_HVControl_Databus) -> Bus Creator/5
  Bus Selector/1 -> Signal Copy/1  "<FL_boCMSleep>"
  Signal Copy/1 -> Bus Creator/2  "OT_boCM_Sleep"
  BDUControl/1(OT_BDUControl_Databus) -> Bus Creator/6
  SystemStatus/1(OT_SystemStatus_Databus) -> Bus Creator/7

== system ChiefMaster_TTC580/ChiefMaster/Flow Logic/BDU Control ==
  FL_BatteryBox_HVControl_Databus : Inport
  FL_KL15_Databus : Inport  Port=2
  IT_Databus : Inport  Port=3
  FL_SystemStatus_Databus : Inport  Port=4
  BDUSystem : Subsystem
      settings: RTWFcnNameOpts=Use subsystem name  RTWFileNameOpts=Use subsystem name
  Bus Creator5 : BusCreator  Inputs=14
  Bus Selector : BusSelector  OutputSignals=FL_boKL15_Disable,FL_boCMSleep
  Bus Selector1 : BusSelector  OutputSignals=IT_UDC_Databus.IT_sUDC_LoadVoltage_V,IT_HW_Input_Databus.IT_boHW_MainHV_Plus_FB,IT_HW_Input_Databus.IT_boHW_MainHV_Minus_FB
  Bus Selector3 : BusSelector  OutputSignals=IT_BatterySignal_Databus.IT_boBMS_HV_REL_ON_BB1,IT_BatterySignal_Databus.IT_boBMS_HV_REL_ON_BB2,IT_BatterySignal_Databus.IT_boBMS_HV_REL_ON_BB3
  Bus Selector4 : BusSelector  OutputSignals=FL_boREQ_HV_ON_BB1,FL_boREQ_HV_ON_BB2,FL_boREQ_HV_ON_BB3
  Bus Selector5 : BusSelector  OutputSignals=FL_boSS_SafeToSD,FL_boSS_System_ESD,FL_boSS_System_SD,FL_sSS_SystemVoltage,FL_boSS_BDU_Reset
  Bus Selector7 : BusSelector  OutputSignals=IT_UDC_Databus.IT_boUDC_SafeToShutdown,IT_UDC_Databus.IT_boUDC_EVDisconnectingDevice,IT_HW_Input_Databus.IT_boHW_DCHV_Plus_FB,IT_HW_Input_Databus.IT_boHW_DCHV_Minus_FB
  Compare To Constant : simulink/Logic and Bit Operations/Compare To Constant  relop===  const=1  OutDataTypeStr=boolean
  NOT : Logic  Operator=NOT  AllPortsSameDT=off  OutDataTypeStr=boolean
  FL_BDUControl_Databus : Outport
  wires:
  Bus Selector3/1 -> BDUSystem/7(IT_boBMS_HV_REL_ON_BB1)  "<IT_boBMS_HV_REL_ON_BB1>"
  Bus Selector3/3 -> BDUSystem/9(IT_boBMS_HV_REL_ON_BB3)  "<IT_boBMS_HV_REL_ON_BB3>"
  Bus Selector3/2 -> BDUSystem/8(IT_boBMS_HV_REL_ON_BB2)  "<IT_boBMS_HV_REL_ON_BB2>"
  Bus Selector4/1 -> BDUSystem/1(FL_boREQ_HV_ON_BB1)  "<FL_boREQ_HV_ON_BB1>"
  Compare To Constant/1 -> NOT/1
  Bus Selector1/2 -> BDUSystem/5(IT_boHW_MainHV_Plus_FB)  "<IT_boHW_MainHV_Plus_FB>"
  Bus Selector1/3 -> BDUSystem/6(IT_boHW_MainHV_Minus_FB)  "<IT_boHW_MainHV_Minus_FB>"
  Bus Selector1/1 -> BDUSystem/4(IT_sUDC_LoadVoltage_V)  "<IT_sUDC_LoadVoltage_V>"
  FL_KL15_Databus/1 -> Bus Selector/1
  Bus Selector/1 -> BDUSystem/19(FL_boKL15_Disable)  "<FL_boKL15_Disable>"
  IT_Databus/1 -> Bus Selector7/1, Bus Selector1/1, Bus Selector3/1
  FL_BatteryBox_HVControl_Databus/1 -> Bus Selector4/1
  Bus Selector4/2 -> BDUSystem/2(FL_boREQ_HV_ON_BB2)  "<FL_boREQ_HV_ON_BB2>"
  Bus Selector4/3 -> BDUSystem/3(FL_boREQ_HV_ON_BB3)  "<FL_boREQ_HV_ON_BB3>"
  BDUSystem/7(FL_boMainHV_Plus_Welded) -> Bus Creator5/7  "FL_boMainHV_Plus_Welded"
  BDUSystem/6(FL_boMainHV_Minus_Welded) -> Bus Creator5/6  "FL_boMainHV_Minus_Welded"
  BDUSystem/5(FL_u8MainHV_Plus_Status) -> Bus Creator5/5  "FL_u8MainHV_Plus_Status"
  BDUSystem/4(FL_u8MainHV_Minus_Status) -> Bus Creator5/4  "FL_u8MainHV_Minus_Status"
  BDUSystem/3(FL_boREQ_MainHV_ON_PLUS) -> Bus Creator5/3  "FL_boREQ_MainHV_ON_PLUS"
  BDUSystem/2(FL_boREQ_MainHV_ON_Precharge) -> Bus Creator5/2  "FL_boREQ_MainHV_ON_Precharge"
  BDUSystem/1(FL_boREQ_MainHV_ON_MINUS) -> Bus Creator5/1  "FL_boREQ_MainHV_ON_MINUS"
  BDUSystem/8(FL_u8Precharge_Status) -> Bus Creator5/8  "FL_u8Precharge_Status"
  Bus Creator5/1 -> FL_BDUControl_Databus/1  "FL_BDUControl_Databus"
  FL_SystemStatus_Databus/1 -> Bus Selector5/1
  Bus Selector5/2 -> BDUSystem/11(FL_boSS_System_ESD)  "<FL_boSS_System_ESD>"
  Bus Selector5/3 -> BDUSystem/12(FL_boSS_System_SD)  "<FL_boSS_System_SD>"
  Bus Selector5/4 -> BDUSystem/13(FL_sSS_SystemVoltage)  "<FL_sSS_SystemVoltage>"
  Bus Selector7/1 -> Compare To Constant/1  "<IT_boUDC_SafeToShutdown>"
  Bus Selector/2 -> BDUSystem/20(FL_boCMSleep)  "<FL_boCMSleep>"
  BDUSystem/9(FL_boMainHV_WeldingCheckActive) -> Bus Creator5/9  "FL_boMainHV_WeldingCheckActive"
  BDUSystem/10(FL_u8WeldingDetection_Status) -> Bus Creator5/10  "FL_u8WeldingDetection_Status"
  NOT/1 -> BDUSystem/15(LoadCurrent)
  Bus Selector5/5 -> BDUSystem/14(FL_boSS_BDU_Reset)  "<FL_boSS_BDU_Reset>"
  Bus Selector7/2 -> BDUSystem/16(IT_boUDC_EVDisconnectingDevice)  "<IT_boUDC_EVDisconnectingDevice>"
  BDUSystem/11(FL_boREQ_DC_ON_MINUS) -> Bus Creator5/11  "FL_boREQ_DC_ON_MINUS"
  BDUSystem/12(FL_boREQ_DC_ON_Plus) -> Bus Creator5/12  "FL_boREQ_DC_ON_Plus"
  Bus Selector5/1 -> BDUSystem/10(FL_boSS_SafeToSD)  "<FL_boSS_SafeToSD>"
  Bus Selector7/3 -> BDUSystem/17(IT_boHW_DCHV_Plus_FB)  "<IT_boHW_DCHV_Plus_FB>"
  Bus Selector7/4 -> BDUSystem/18(IT_boHW_DCHV_Minus_FB)  "<IT_boHW_DCHV_Minus_FB>"
  BDUSystem/13(FL_u8DCHV_Minus_Status) -> Bus Creator5/13
  BDUSystem/14(FL_u8DCHV_Plus_Status) -> Bus Creator5/14

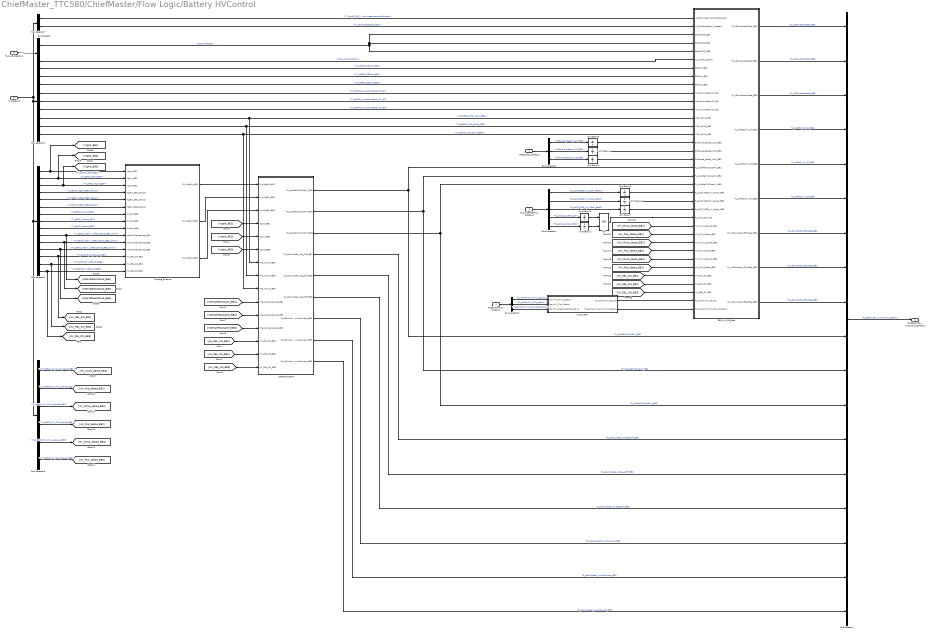
== system ChiefMaster_TTC580/ChiefMaster/Flow Logic/Battery HVControl ==
  Reset_Req_Databus : Inport
  FL_KL15_Databus : Inport  Port=2
  IT_Databus : Inport  Port=3
  FL_BDUControl_Databus : Inport  Port=4
  FL_SystemStatus_Databus : Inport  Port=5
  Bus Creator4 : BusCreator  Inputs=18
  Bus Selector : BusSelector  OutputSignals=FL_boCMSleep,FL_boKL15_Disable
  Bus Selector1 : BusSelector  OutputSignals=IT_BatterySignal_Databus.IT_boBMS_SDError_BB1,IT_BatterySignal_Databus.IT_boBMS_SDError_BB2,IT_BatterySignal_Databus.IT_boBMS_SDError_BB3,IT_BatterySignal_Databus.IT_boBMS_InsulationReadyOK_B1,IT_BatterySignal_Databus.IT_boBMS_InsulationReadyOK_B2,IT_BatterySignal_Databus.IT_boBMS_InsulationReadyOK_B3,IT_BatterySignal_Databus.IT_boBMS_IMD_Active_BB1,IT_BatterySignal_Databus.IT_boBMS_IMD_Active_BB2,IT_BatterySignal_Databus.IT_boBMS_IMD_Active_BB3
  Bus Selector2 : BusSelector  OutputSignals=IT_BatterySignal_Databus.IT_sBMS_VtgInt_BB1,IT_BatterySignal_Databus.IT_sBMS_VtgInt_BB2,IT_BatterySignal_Databus.IT_sBMS_VtgInt_BB3,IT_BatterySignal_Databus.IT_sBMS_VtgExt_BB1_Sensor,IT_BatterySignal_Databus.IT_sBMS_VtgExt_BB2_Sensor,IT_BatterySignal_Databus.IT_sBMS_VtgExt_BB3_Sensor,IT_BatterySignal_Databus.IT_sBMS_Current_BB1,IT_BatterySignal_Databus.IT_sBMS_Current_BB2,IT_BatterySignal_Databus.IT_sBMS_Current_BB3,IT_BatterySignal_Databus.IT_sBMS_InternalResistance_BB1_ohms,IT_BatterySignal_Databus.IT_sBMS_InternalResistance_BB2_ohms,IT_BatterySignal_Databus.IT_sBMS_InternalResistance_BB3_ohms,IT_BatterySignal_Databus.IT_boBMS_HV_REL_ON_BB1,IT_BatterySignal_Databus.IT_boBMS_HV_REL_ON_BB2,IT_BatterySignal_Databus.IT_boBMS_HV_REL_ON_BB3
  Bus Selector3 : BusSelector  OutputSignals=IT_BatterySignal_Databus.IT_boBMS_HV_Minus_Sense_BB1,IT_BatterySignal_Databus.IT_boBMS_HV_Plus_Sense_BB1,IT_BatterySignal_Databus.IT_boBMS_HV_Minus_Sense_BB2,IT_BatterySignal_Databus.IT_boBMS_HV_Plus_Sense_BB2,IT_BatterySignal_Databus.IT_boBMS_HV_Minus_Sense_BB3,IT_BatterySignal_Databus.IT_boBMS_HV_Plus_Sense_BB3
  Bus Selector4 : BusSelector  OutputSignals=FL_boSS_REQ_HV_Open_Batt1,FL_boSS_REQ_HV_Open_Batt2,FL_boSS_REQ_HV_Open_Batt3,FL_boSS_System_SD,FL_boSS_System_ESD
  Bus Selector5 : BusSelector  OutputSignals=FL_u8MainHV_Minus_Status,FL_u8MainHV_Plus_Status,FL_boMainHV_WeldingCheckActive
  Bus Selector6 : BusSelector  OutputSignals=Software_Reset_KL15_BB1,Software_Reset_KL15_BB2,Software_Reset_KL15_BB3
  Bus Selector7 : BusSelector  OutputSignals=IT_UDC_Databus.IT_boUDC_EV_IsolationMeasurementRequest,IT_UDC_Databus.IT_boChargeStop_Button
  OR : Logic  Operator=OR  AllPortsSameDT=off  OutDataTypeStr=boolean
  REQ_HV_ON_Batt : Subsystem  TreatAsAtomicUnit=on
      settings: RTWFcnNameOpts=Use subsystem name  RTWFileNameOpts=Use subsystem name
  SafeToCloseHV : Subsystem  TreatAsAtomicUnit=on
      settings: RTWFcnNameOpts=Use subsystem name  RTWFileNameOpts=Use subsystem name
  Subsystem : Subsystem
  Unit Delay{1..7,9} (8 alike) : UnitDelay  SampleTime=-1  HasFrameUpgradeWarning=on
  Voltage_External : Subsystem
      settings: RTWFcnNameOpts=Use subsystem name  RTWFileNameOpts=Use subsystem name
  FL_BatteryBox_HVControl_Databus : Outport
  wires:
  FL_SystemStatus_Databus/1 -> Bus Selector4/1
  SafeToCloseHV/1(FL_boSafeToCloseHV_BB1) -> REQ_HV_ON_Batt/19(FL_boSafeToCloseHV_BB1), Bus Creator4/10  "FL_boSafeToCloseHV_BB1"
  Bus Selector/1 -> REQ_HV_ON_Batt/3(SafeToSD_BB1), REQ_HV_ON_Batt/4(SafeToSD_BB2), REQ_HV_ON_Batt/5(SafeToSD_BB3)  "<FL_boCMSleep>"
  Voltage_External/3(FL_sVtgExt_BB3) -> SafeToCloseHV/3(FL_sVtgExt_BB3)
  Bus Selector1/2 -> REQ_HV_ON_Batt/8(SDError_BB2)  "<IT_boBMS_SDError_BB2>"
  Voltage_External/2(FL_sVtgExt_BB2) -> SafeToCloseHV/2(FL_sVtgExt_BB2)
  Unit Delay9/1 -> OR/1
  SafeToCloseHV/2(FL_boSafeToCloseHV_BB2) -> REQ_HV_ON_Batt/20(FL_boSafeToCloseHV_BB2), Bus Creator4/11  "FL_boSafeToCloseHV_BB2"
  Voltage_External/1(FL_sVtgExt_BB1) -> SafeToCloseHV/1(FL_sVtgExt_BB1)
  Bus Selector/2 -> REQ_HV_ON_Batt/6(KL15_CM_disable)  "<FL_boKL15_Disable>"
  Bus Selector6/3 -> Unit Delay3/1  "<Software_Reset_KL15_BB3>"
  Bus Selector6/1 -> Unit Delay5/1  "<Software_Reset_KL15_BB1>"
  Bus Selector1/3 -> REQ_HV_ON_Batt/9(SDError_BB3)  "<IT_boBMS_SDError_BB3>"
  Bus Selector6/2 -> Unit Delay4/1  "<Software_Reset_KL15_BB2>"
  SafeToCloseHV/3(FL_boSafeToCloseHV_BB3) -> REQ_HV_ON_Batt/21(FL_boSafeToCloseHV_BB3), Bus Creator4/12  "FL_boSafeToCloseHV_BB3"
  Bus Selector1/1 -> REQ_HV_ON_Batt/7(SDError_BB1)  "<IT_boBMS_SDError_BB1>"
  [HV_Minus_Sense_BB1] -> REQ_HV_ON_Batt/26(HV_Minus_Sense_BB1)
  [HV_Plus_Sense_BB1] -> REQ_HV_ON_Batt/27(HV_Plus_Sense_BB1)
  [HV_Minus_Sense_BB2] -> REQ_HV_ON_Batt/28(HV_Minus_Sense_BB2)
  [HV_Plus_Sense_BB2] -> REQ_HV_ON_Batt/29(HV_Plus_Sense_BB2)
  [HV_Minus_Sense_BB3] -> REQ_HV_ON_Batt/30(HV_Minus_Sense_BB3)
  [HV_Plus_Sense_BB3] -> REQ_HV_ON_Batt/31(HV_Plus_Sense_BB3)
  [HV_REL_ON_BB2] -> REQ_HV_ON_Batt/33(HV_REL_ON_BB1)
  [HV_REL_ON_BB3] -> REQ_HV_ON_Batt/34(HV_REL_ON_BB3)
  [HV_REL_ON_BB1] -> REQ_HV_ON_Batt/32(HV_REL_ON_BB2)
  Subsystem/1(FL_boMainHV_SD_OK) -> REQ_HV_ON_Batt/35(FL_boMainHV_SD_OK)
  FL_KL15_Databus/1 -> Bus Selector/1
  IT_Databus/1 -> Bus Selector3/1, Bus Selector2/1, Bus Selector1/1, Bus Selector7/1
  Bus Selector1/4 -> REQ_HV_ON_Batt/10(InsulationReadyOK_B1)  "<IT_boBMS_InsulationReadyOK_B1>"
  Bus Selector1/5 -> REQ_HV_ON_Batt/11(InsulationReadyOK_B2)  "<IT_boBMS_InsulationReadyOK_B2>"
  Bus Selector1/6 -> REQ_HV_ON_Batt/12(InsulationReadyOK_B3)  "<IT_boBMS_InsulationReadyOK_B3>"
  Bus Selector1/7 -> SafeToCloseHV/7(IMD_Active_BB1), REQ_HV_ON_Batt/13(IMD_Active_BB1)  "<IT_boBMS_IMD_Active_BB1>"
  Bus Selector1/8 -> SafeToCloseHV/8(IMD_Active_BB2), REQ_HV_ON_Batt/14(IMD_Active_BB2)  "<IT_boBMS_IMD_Active_BB2>"
  Bus Selector1/9 -> SafeToCloseHV/9(IMD_Active_BB3), REQ_HV_ON_Batt/15(IMD_Active_BB3)  "<IT_boBMS_IMD_Active_BB3>"
  Bus Selector2/4 -> Voltage_External/4(VtgExt_BB1_Sensor)  "<IT_sBMS_VtgExt_BB1_Sensor>"
  Bus Selector2/5 -> Voltage_External/5(VtgExt_BB2_Sensor)  "<IT_sBMS_VtgExt_BB2_Sensor>"
  Bus Selector2/6 -> Voltage_External/6(VtgExt_BB3_Sensor)  "<IT_sBMS_VtgExt_BB3_Sensor>"
  Bus Selector2/1 -> Voltage_External/1(VtgInt_BB1), [VtgInt_BB1]  "<IT_sBMS_VtgInt_BB1>"
  Bus Selector2/2 -> Voltage_External/2(VtgInt_BB2), [VtgInt_BB2]  "<IT_sBMS_VtgInt_BB2>"
  Bus Selector2/3 -> Voltage_External/3(VtgInt_BB3), [VtgInt_BB3]  "<IT_sBMS_VtgInt_BB3>"
  Bus Selector2/10 -> Voltage_External/10(InternalResistance_BB1), [InternalResistance_BB1]  "<IT_sBMS_InternalResistance_BB1_ohms>"
  Bus Selector2/11 -> Voltage_External/11(InternalResistance_BB2), [InternalResistance_BB2]  "<IT_sBMS_InternalResistance_BB2_ohms>"
  Bus Selector2/12 -> Voltage_External/12(InternalResistance_BB3), [InternalResistance_BB3]  "<IT_sBMS_InternalResistance_BB3_ohms>"
  Bus Selector2/7 -> Voltage_External/7(Current_BB1)  "<IT_sBMS_Current_BB1>"
  Bus Selector2/8 -> Voltage_External/8(Current_BB2)  "<IT_sBMS_Current_BB2>"
  Bus Selector2/9 -> Voltage_External/9(Current_BB3)  "<IT_sBMS_Current_BB3>"
  Bus Selector2/13 -> Voltage_External/13(HV_REL_ON_BB1), [HV_REL_ON_BB1]  "<IT_boBMS_HV_REL_ON_BB1>"
  Bus Selector2/14 -> Voltage_External/14(HV_REL_ON_BB2), [HV_REL_ON_BB2]  "<IT_boBMS_HV_REL_ON_BB2>"
  Bus Selector2/15 -> Voltage_External/15(HV_REL_ON_BB3), [HV_REL_ON_BB3]  "<IT_boBMS_HV_REL_ON_BB3>"
  [VtgInt_BB1] -> SafeToCloseHV/4(VtgInt_BB1)
  [VtgInt_BB2] -> SafeToCloseHV/5(VtgInt_BB2)
  [VtgInt_BB3] -> SafeToCloseHV/6(VtgInt_BB3)
  [InternalResistance_BB1] -> SafeToCloseHV/10(InternalResistance_BB1)
  [InternalResistance_BB2] -> SafeToCloseHV/11(InternalResistance_BB2)
  [InternalResistance_BB3] -> SafeToCloseHV/12(InternalResistance_BB3)
  Bus Selector3/1 -> [HV_Minus_Sense_BB1]  "<IT_boBMS_HV_Minus_Sense_BB1>"
  Bus Selector3/2 -> [HV_Plus_Sense_BB1]  "<IT_boBMS_HV_Plus_Sense_BB1>"
  Bus Selector3/3 -> [HV_Minus_Sense_BB2]  "<IT_boBMS_HV_Minus_Sense_BB2>"
  Bus Selector3/4 -> [HV_Plus_Sense_BB2]  "<IT_boBMS_HV_Plus_Sense_BB2>"
  Bus Selector3/5 -> [HV_Minus_Sense_BB3]  "<IT_boBMS_HV_Minus_Sense_BB3>"
  Bus Selector3/6 -> [HV_Plus_Sense_BB3]  "<IT_boBMS_HV_Plus_Sense_BB3>"
  Bus Selector4/4 -> Unit Delay9/1  "<FL_boSS_System_SD>"
  FL_BDUControl_Databus/1 -> Bus Selector5/1
  Reset_Req_Databus/1 -> Bus Selector6/1
  REQ_HV_ON_Batt/5(FL_boREQ_HV_ON_BB2) -> Bus Creator4/5  "FL_boREQ_HV_ON_BB2"
  REQ_HV_ON_Batt/4(FL_boREQ_HV_ON_BB1) -> Bus Creator4/4  "FL_boREQ_HV_ON_BB1"
  REQ_HV_ON_Batt/6(FL_boREQ_HV_ON_BB3) -> Bus Creator4/6  "FL_boREQ_HV_ON_BB3"
  REQ_HV_ON_Batt/3(FL_u8ContactorState_BB3) -> Bus Creator4/3  "FL_u8ContactorState_BB3"
  REQ_HV_ON_Batt/7(FL_u8Contactor_FB_State_BB1) -> Bus Creator4/7  "FL_u8Contactor_FB_State_BB1"
  REQ_HV_ON_Batt/2(FL_u8ContactorState_BB2) -> Bus Creator4/2  "FL_u8ContactorState_BB2"
  REQ_HV_ON_Batt/8(FL_u8Contactor_FB_State_BB2) -> Bus Creator4/8  "FL_u8Contactor_FB_State_BB2"
  REQ_HV_ON_Batt/1(FL_u8ContactorState_BB1) -> Bus Creator4/1  "FL_u8ContactorState_BB1"
  REQ_HV_ON_Batt/9(FL_u8Contactor_FB_State_BB3) -> Bus Creator4/9  "FL_u8Contactor_FB_State_BB3"
  Bus Creator4/1 -> FL_BatteryBox_HVControl_Databus/1  "FL_BatteryBox_HVControl_Databus"
  Bus Selector5/1 -> Subsystem/1(MainHV_Minus_Status)  "<FL_u8MainHV_Minus_Status>"
  Bus Selector5/2 -> Subsystem/2(MainHV_Plus_Status)  "<FL_u8MainHV_Plus_Status>"
  Bus Selector4/5 -> Unit Delay1/1  "<FL_boSS_System_ESD>"
  Unit Delay1/1 -> OR/2
  OR/1 -> REQ_HV_ON_Batt/25(FL_boSystem_SD)
  Bus Selector5/3 -> Subsystem/3(MainHV_WeldingCheckActive)  "<FL_boMainHV_WeldingCheckActive>"
  [HV_REL_ON_BB1] -> SafeToCloseHV/13(HV_REL_ON_BB1)
  [HV_REL_ON_BB2] -> SafeToCloseHV/14(HV_REL_ON_BB2)
  [HV_REL_ON_BB3] -> SafeToCloseHV/15(HV_REL_ON_BB3)
  SafeToCloseHV/4(FL_sCalculated_Vtg_Diff_BB1) -> Bus Creator4/13  "FL_sCalculated_VoltageDiff_BB1"
  SafeToCloseHV/5(FL_sCalculated_Vtg_Diff_BB2) -> Bus Creator4/14  "FL_sCalculated_VoltageDiff_BB2"
  SafeToCloseHV/6(FL_sCalculated_Vtg_Diff_BB3) -> Bus Creator4/15  "FL_sCalculated_VoltageDiff_BB3"
  SafeToCloseHV/7(FL_sCalculated_InrushCurrent_BB1) -> Bus Creator4/16  "FL_sCalculated_InrushCurrent_BB1"
  SafeToCloseHV/8(FL_sCalculated_InrushCurrent_BB2) -> Bus Creator4/17  "FL_sCalculated_InrushCurrent_BB2"
  SafeToCloseHV/9(FL_sCalculated_InrushCurrent_BB3) -> Bus Creator4/18  "FL_sCalculated_InrushCurrent_BB3"
  Subsystem/2(FL_boMainHV_PlusMinus_Status) -> REQ_HV_ON_Batt/36(FL_boMainHV_PlusMinus_Status)
  Unit Delay3/1 -> REQ_HV_ON_Batt/18(Software_Reset_KL15_BB1)
  Unit Delay4/1 -> REQ_HV_ON_Batt/17(Software_Reset_KL15_BB2)
  Unit Delay5/1 -> REQ_HV_ON_Batt/16(Software_Reset_KL15_BB3)
  Bus Selector4/1 -> Unit Delay2/1  "<FL_boSS_REQ_HV_Open_Batt1>"
  Bus Selector4/2 -> Unit Delay6/1  "<FL_boSS_REQ_HV_Open_Batt2>"
  Bus Selector4/3 -> Unit Delay7/1  "<FL_boSS_REQ_HV_Open_Batt3>"
  Unit Delay2/1 -> REQ_HV_ON_Batt/22(FL_boST_REQ_HV_Open_BB1)
  Unit Delay6/1 -> REQ_HV_ON_Batt/23(FL_boST_REQ_HV_Open_BB2)
  Unit Delay7/1 -> REQ_HV_ON_Batt/24(FL_boST_REQ_HV_Open_BB3)
  Bus Selector7/1 -> REQ_HV_ON_Batt/1(IsolationMeasurementRequest)  "<IT_boUDC_EV_IsolationMeasurementRequest>"
  Bus Selector7/2 -> REQ_HV_ON_Batt/2(IP_boChargeStop_Pressed)  "<IT_boChargeStop_Button>"

== system ChiefMaster_TTC580/ChiefMaster/Flow Logic/IMD Control ==
  IT_Databus : Inport
  FL_SystemStatus_Databus : Inport  Port=2
  Bus Creator2 : BusCreator  Inputs=6
  Bus Selector1 : BusSelector  OutputSignals=IT_UDC_Databus.IT_boUDC_KL15_D,IT_UDC_Databus.IT_boUDC_KL15_C,IT_BatterySignal_Databus.IT_boBMS_HV_ON_BB,IT_BatterySignal_Databus.IT_u8BMS_BB_No_MaxVoltage,IT_BatterySignal_Databus.IT_u8BMS_BB_No_MinVoltage,IT_BatterySignal_Databus.IT_boBMS_SDError_BB1,IT_BatterySignal_Databus.IT_boBMS_SDError_BB2,IT_BatterySignal_Databus.IT_boBMS_SDError_BB3,IT_BatterySignal_Databus.IT_boBMS_InsulationReadyOK_B1,IT_BatterySignal_Databus.IT_boBMS_InsulationReadyOK_B2,IT_BatterySignal_Databus.IT_boBMS_InsulationReadyOK_B3,IT_BatterySignal_Databus.IT_boBMS_IMD_Active_BB1,IT_BatterySignal_Databus.IT_boBMS_IMD_Active_BB2,IT_BatterySignal_Databus.IT_boBMS_IMD_Active_BB3,IT_BatterySignal_Databus.IT_boBMS_HV_REL_ON_BB1,IT_BatterySignal_Databus.IT_boBMS_HV_REL_ON_BB2,IT_BatterySignal_Databus.IT_boBMS_HV_REL_ON_BB3,IT_BatterySignal_Databus.IT_boBMS_Batt1_Availability,IT_BatterySignal_Databus.IT_boBMS_Batt2_Availability,IT_BatterySignal_Databus.IT_boBMS_Batt3_Availability,IT_UDC_Databus.IT_boUDC_EV_IsolationMeasurementRequest
  Bus Selector2 : BusSelector  OutputSignals=FL_boSS_System_SD,FL_boSS_System_ESD
  InsulationMonitoringReq : Subsystem  TreatAsAtomicUnit=on
      settings: RTWFcnNameOpts=Use subsystem name  RTWFileNameOpts=Use subsystem name
  FL_IMD_Control_Databus : Outport
  wires:
  Bus Selector1/10 -> InsulationMonitoringReq/10(IT_boBMS_InsulationReadyOK_B2)  "<IT_boBMS_InsulationReadyOK_B2>"
  Bus Selector1/4 -> InsulationMonitoringReq/4(<IT_u8BMS_BB_No_MaxVoltage>)  "<IT_u8BMS_BB_No_MaxVoltage>"
  Bus Selector1/9 -> InsulationMonitoringReq/9(IT_boBMS_InsulationReadyOK_B1)  "<IT_boBMS_InsulationReadyOK_B1>"
  Bus Selector1/5 -> InsulationMonitoringReq/5(<IT_u8BMS_BB_No_MinVoltage>)  "<IT_u8BMS_BB_No_MinVoltage>"
  InsulationMonitoringReq/1(FL_boREQ_IMD_ON_BB1) -> Bus Creator2/1
  Bus Selector1/3 -> InsulationMonitoringReq/3(IT_boBMS_HV_ON_BB)  "<IT_boBMS_HV_ON_BB>"
  Bus Selector1/7 -> InsulationMonitoringReq/7(IT_boBMS_SDError_BB2)  "<IT_boBMS_SDError_BB2>"
  Bus Selector1/11 -> InsulationMonitoringReq/11(IT_boBMS_InsulationReadyOK_B3)  "<IT_boBMS_InsulationReadyOK_B3>"
  Bus Selector1/8 -> InsulationMonitoringReq/8(IT_boBMS_SDError_BB3)  "<IT_boBMS_SDError_BB3>"
  Bus Selector1/6 -> InsulationMonitoringReq/6(IT_boBMS_SDError_BB1)  "<IT_boBMS_SDError_BB1>"
  InsulationMonitoringReq/3(FL_boREQ_IMD_ON_BB3) -> Bus Creator2/3
  InsulationMonitoringReq/2(FL_boREQ_IMD_ON_BB2) -> Bus Creator2/2
  Bus Selector1/13 -> InsulationMonitoringReq/13(IT_boBMS_IMD_Active_BB2)  "<IT_boBMS_IMD_Active_BB2>"
  IT_Databus/1 -> Bus Selector1/1
  Bus Creator2/1 -> FL_IMD_Control_Databus/1  "FL_IMD_Control_Databus"
  Bus Selector1/15 -> InsulationMonitoringReq/15(IT_boBMS_HV_REL_ON_BB1)  "<IT_boBMS_HV_REL_ON_BB1>"
  Bus Selector1/16 -> InsulationMonitoringReq/16(IT_boBMS_HV_REL_ON_BB2)  "<IT_boBMS_HV_REL_ON_BB2>"
  Bus Selector1/17 -> InsulationMonitoringReq/17(IT_boBMS_HV_REL_ON_BB3)  "<IT_boBMS_HV_REL_ON_BB3>"
  FL_SystemStatus_Databus/1 -> Bus Selector2/1
  Bus Selector1/1 -> InsulationMonitoringReq/1(IT_boUDC_KL15_D)  "<IT_boUDC_KL15_D>"
  Bus Selector1/2 -> InsulationMonitoringReq/2(IT_boUDC_KL15_C)  "<IT_boUDC_KL15_C>"
  Bus Selector2/1 -> InsulationMonitoringReq/22(FL_boSS_System_SD)  "<FL_boSS_System_SD>"
  Bus Selector2/2 -> InsulationMonitoringReq/23(FL_boSS_System_ESD)  "<FL_boSS_System_ESD>"
  Bus Selector1/18 -> InsulationMonitoringReq/18(IT_sBMS_Batt1_Availability)  "<IT_boBMS_Batt1_Availability>"
  Bus Selector1/19 -> InsulationMonitoringReq/19(IT_sBMS_Batt2_Availability)  "<IT_boBMS_Batt2_Availability>"
  Bus Selector1/20 -> InsulationMonitoringReq/20(IT_sBMS_Batt3_Availability)  "<IT_boBMS_Batt3_Availability>"
  Bus Selector1/12 -> InsulationMonitoringReq/12(IT_boBMS_IMD_Active_BB1)  "<IT_boBMS_IMD_Active_BB1>"
  Bus Selector1/14 -> InsulationMonitoringReq/14(IT_boBMS_IMD_Active_BB3)  "<IT_boBMS_IMD_Active_BB3>"
  Bus Selector1/21 -> InsulationMonitoringReq/21(IT_boUDC_EV_IsolationMeasurementRequest)  "<IT_boUDC_EV_IsolationMeasurementRequest>"
  InsulationMonitoringReq/4(FL_u8_IMD_State_BB1) -> Bus Creator2/4
  InsulationMonitoringReq/5(FL_u8_IMD_State_BB2) -> Bus Creator2/5
  InsulationMonitoringReq/6(FL_u8_IMD_State_BB3) -> Bus Creator2/6

== system ChiefMaster_TTC580/ChiefMaster/Flow Logic/KL15 ==
  IT_Databus : Inport
  FL_BatteryBox_HVControl_Databus : Inport  Port=2
  Reset_Req_Databus : Inport  Port=3
  Bus Creator : BusCreator  Inputs=6
  Bus Selector : BusSelector  OutputSignals=Software_Reset_KL15_BB1,Software_Reset_KL15_BB2,Software_Reset_KL15_BB3
  Bus Selector1 : BusSelector  OutputSignals=FL_u8Contactor_FB_State_BB1,FL_u8Contactor_FB_State_BB2,FL_u8Contactor_FB_State_BB3
  Bus Selector2 : BusSelector  OutputSignals=IT_HW_Input_Databus.IT_boHW_KL15,IT_UDC_Databus.IT_boUDC_KL15_D,IT_UDC_Databus.IT_boUDC_KL15_C
  System_KL15 : Subsystem
      settings: RTWFcnNameOpts=Use subsystem name  RTWFileNameOpts=Use subsystem name
  Unit Delay{,1..2,6..8} (6 alike) : UnitDelay  SampleTime=-1  HasFrameUpgradeWarning=on
  FL_KL15_Databus : Outport
  wires:
  Unit Delay1/1 -> System_KL15/5(Reset_BB2)
  Bus Selector1/2 -> Unit Delay7/1  "<FL_u8Contactor_FB_State_BB2>"
  Bus Selector1/3 -> Unit Delay8/1  "<FL_u8Contactor_FB_State_BB3>"
  Unit Delay8/1 -> System_KL15/9(Contactor_FB_State_BB3)
  Unit Delay7/1 -> System_KL15/8(Contactor_FB_State_BB2)
  Unit Delay6/1 -> System_KL15/7(Contactor_FB_State_BB1)
  Bus Selector1/1 -> Unit Delay6/1  "<FL_u8Contactor_FB_State_BB1>"
  Unit Delay/1 -> System_KL15/4(Reset_BB1)
  Unit Delay2/1 -> System_KL15/6(Reset_BB3)
  System_KL15/4(FL_boKL15_BB3) -> Bus Creator/4
  System_KL15/2(FL_boKL15_BB1) -> Bus Creator/2
  System_KL15/3(FL_boKL15_BB2) -> Bus Creator/3
  System_KL15/5(FL_boKL15_Disable) -> Bus Creator/5
  System_KL15/6(FL_boKL15_Reset) -> Bus Creator/6
  Bus Creator/1 -> FL_KL15_Databus/1  "FL_KL15_Databus"
  Reset_Req_Databus/1 -> Bus Selector/1
  FL_BatteryBox_HVControl_Databus/1 -> Bus Selector1/1
  Bus Selector/1 -> Unit Delay/1  "<Software_Reset_KL15_BB1>"
  Bus Selector/2 -> Unit Delay1/1  "<Software_Reset_KL15_BB2>"
  Bus Selector/3 -> Unit Delay2/1  "<Software_Reset_KL15_BB3>"
  System_KL15/1(FL_boCMSleep) -> Bus Creator/1
  IT_Databus/1 -> Bus Selector2/1
  Bus Selector2/1 -> System_KL15/1(IT_boHW_KL15)  "<IT_boHW_KL15>"
  Bus Selector2/2 -> System_KL15/2(IT_boUDC_KL15_D)  "<IT_boUDC_KL15_D>"
  Bus Selector2/3 -> System_KL15/3(IT_boUDC_KL15_C)  "<IT_boUDC_KL15_C>"

== system ChiefMaster_TTC580/ChiefMaster/Flow Logic/Reset ==
  FL_KL15_Databus : Inport
  IT_Databus : Inport  Port=2
  FL_BatteryBox_HVControl_Databus : Inport  Port=3
  Bus Creator3 : BusCreator  Inputs=5
  Bus Selector : BusSelector  OutputSignals=FL_boKL15_BB1,FL_boKL15_BB2,FL_boKL15_BB3
  Bus Selector1 : BusSelector  OutputSignals=IT_UDC_Databus.IT_boUDC_KL15_C,IT_UDC_Databus.IT_boUDC_KL15_D,IT_BatterySignal_Databus.IT_u8BMS_BB_No_MaxVoltage,IT_BatterySignal_Databus.IT_u8BMS_BB_No_MinVoltage,IT_BatterySignal_Databus.IT_boBMS_SDError_BB1,IT_BatterySignal_Databus.IT_boBMS_SDError_BB2,IT_BatterySignal_Databus.IT_boBMS_SDError_BB3
  Bus Selector2 : BusSelector  OutputSignals=FL_u8ContactorState_BB1,FL_u8ContactorState_BB2,FL_u8ContactorState_BB3
  Reset_Req : Subsystem
      settings: RTWFcnNameOpts=Use subsystem name  RTWFileNameOpts=Use subsystem name
  FL_ResetReq_Databus : Outport
  wires:
  Bus Selector/2 -> Reset_Req/2(KL_15_BB2)  "<FL_boKL15_BB2>"
  Reset_Req/3(Software_Reset_KL15_BB3) -> Bus Creator3/3
  Reset_Req/5(Software_Reset_KL15_ALL) -> Bus Creator3/5
  Reset_Req/1(Software_Reset_KL15_BB1) -> Bus Creator3/1
  Bus Selector1/7 -> Reset_Req/10(SDError_BB3)  "<IT_boBMS_SDError_BB3>"
  Bus Selector/1 -> Reset_Req/1(KL_15_BB1)  "<FL_boKL15_BB1>"
  Reset_Req/4(Manual_Reset_KL15_ALL) -> Bus Creator3/4
  Bus Selector1/2 -> Reset_Req/5(DriveMode)  "<IT_boUDC_KL15_D>"
  Bus Selector1/5 -> Reset_Req/8(SDError_BB1)  "<IT_boBMS_SDError_BB1>"
  Bus Selector1/1 -> Reset_Req/4(ChargeMode)  "<IT_boUDC_KL15_C>"
  Bus Selector/3 -> Reset_Req/3(KL_15_BB3)  "<FL_boKL15_BB3>"
  Bus Selector1/4 -> Reset_Req/7(MinVtgBB)  "<IT_u8BMS_BB_No_MinVoltage>"
  Bus Selector1/3 -> Reset_Req/6(MaxVtgBB)  "<IT_u8BMS_BB_No_MaxVoltage>"
  Reset_Req/2(Software_Reset_KL15_BB2) -> Bus Creator3/2
  FL_KL15_Databus/1 -> Bus Selector/1
  IT_Databus/1 -> Bus Selector1/1
  Bus Creator3/1 -> FL_ResetReq_Databus/1  "FL_ResetReq_Databus"
  FL_BatteryBox_HVControl_Databus/1 -> Bus Selector2/1
  Bus Selector2/1 -> Reset_Req/11(ContactorState_BB1)  "<FL_u8ContactorState_BB1>"
  Bus Selector2/2 -> Reset_Req/12(ContactorState_BB2)  "<FL_u8ContactorState_BB2>"
  Bus Selector2/3 -> Reset_Req/13(ContactorState_BB3)  "<FL_u8ContactorState_BB3>"
  Bus Selector1/6 -> Reset_Req/9(SDError_BB2)  "<IT_boBMS_SDError_BB2>"
